simulink model "SistemaTotal"  (R2014b)
settings: Solver=FixedStepDiscrete  StartTime=0.0  StopTime=3000  RelTol=1e-3
undefined symbols (not defined in the file): M, T
settings Model: CovSFcnEnable=on  Creator=Afonso  LastModifiedBy=alunos
settings OptimizationCC: UseDivisionForNetSlopeComputation=off  SimCompilerOptimization=off
settings DebuggingCC: SolverPrmCheckMsg=none  FrameProcessingCompatibilityMsg=error
settings RTWCC: RTWCompilerOptimization=off

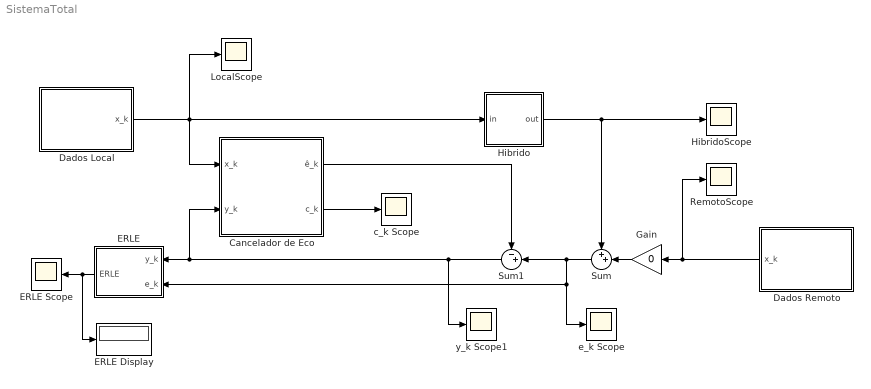
== system SistemaTotal ==
  Cancelador de Eco : Subsystem
  Dados Local : Subsystem
  Dados Remoto : Subsystem
  ERLE : Subsystem
  ERLE Display : Display
  ERLE Scope : Scope
      settings: TimeRange=1400  YMin=-1000  YMax=200  SaveName=ERLE
  Gain : Gain  Gain=0
  Hibrido : Subsystem
  HibridoScope : Scope
      settings: SaveName=Hibrido
  LocalScope : Scope
      settings: SaveName=Local
  RemotoScope : Scope
      settings: SaveName=Remoto
  Sum : Sum  Inputs=++|
  Sum1 : Sum  Inputs=-+|
  "c_k Scope " : Scope
      settings: SaveName=Coeficientes
  e_k Scope : Scope
      settings: SaveName=Eco
  y_k Scope1 : Scope
      settings: SaveName=Erro
  wires:
  Dados Local/1(x_k) -> LocalScope/1, Hibrido/1(in), Cancelador de Eco/1(x_k)
  Dados Remoto/1(x_k) -> RemotoScope/1, Gain/1
  Gain/1 -> Sum/2
  Hibrido/1(out) -> HibridoScope/1, Sum/1
  Cancelador de Eco/1(ê_k) -> Sum1/1
  ERLE/1(ERLE) -> ERLE Display/1, ERLE Scope/1
  Sum/1 -> e_k Scope/1, ERLE/2(e_k), Sum1/2
  Sum1/1 -> y_k Scope1/1, Cancelador de Eco/2(y_k), ERLE/1(y_k)
  Cancelador de Eco/2(c_k) -> "c_k Scope "/1

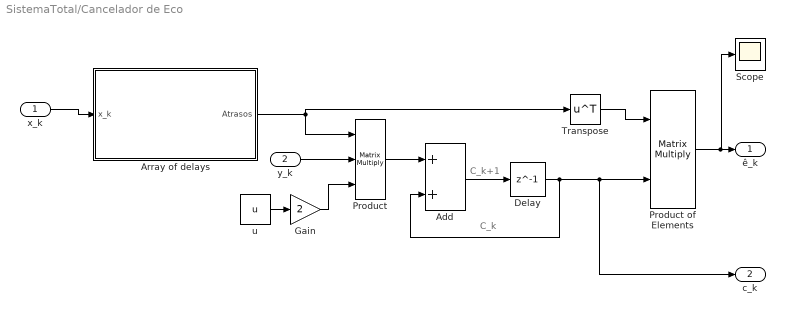
== system SistemaTotal/Cancelador de Eco ==
  note: C_k
  note: C_k+1
  x_k : Inport
  y_k : Inport  Port=2
  Add : Sum
  Array of delays : Subsystem
  Delay : Delay  DelayLength=1  SampleTime=T
  Gain : Gain  Gain=2
  Product : Product  Inputs=3  Multiplication=Matrix(*)
  Product of Elements : Product  Inputs=**  Multiplication=Matrix(*)
  Scope : Scope
  Transpose : Math  Operator=transpose  SaturateOnIntegerOverflow=on
  u : Constant  Value=u  SampleTime=T
  ê_k : Outport
  c_k : Outport  Port=2
  wires:
  y_k/1 -> Product/2
  u/1 -> Gain/1
  Gain/1 -> Product/3
  x_k/1 -> Array of delays/1(x_k)
  Product/1 -> Add/1
  Product of Elements/1 -> ê_k/1, Scope/1
  Add/1 -> Delay/1
  Delay/1 -> c_k/1, Product of Elements/2, Add/2
  Transpose/1 -> Product of Elements/1
  Array of delays/1(Atrasos) -> Product/1, Transpose/1

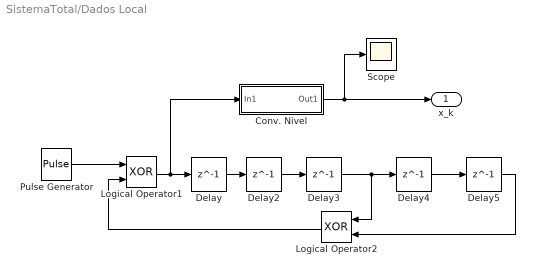
== system SistemaTotal/Dados Local ==
  Conv. Nivel : Subsystem
  Delay : Delay  DelayLength=1  SampleTime=T
  Delay{2..5} (4 alike) : Delay  DelayLength=1
  Logical Operator1 : Logic  Operator=XOR  AllPortsSameDT=off  OutDataTypeStr=boolean
  Logical Operator2 : Logic  Operator=XOR  AllPortsSameDT=off  OutDataTypeStr=boolean
  Pulse Generator : DiscretePulseGenerator  PulseType=Time based  Period=2*T  PulseWidth=50
  Scope : Scope
      settings: YMin=-1.5  YMax=1.5
  x_k : Outport
  wires:
  Delay2/1 -> Delay3/1
  Delay/1 -> Delay2/1
  Delay4/1 -> Delay5/1
  Delay3/1 -> Logical Operator2/1, Delay4/1
  Logical Operator2/1 -> Logical Operator1/2
  Delay5/1 -> Logical Operator2/2
  Logical Operator1/1 -> Conv. Nivel/1(In1), Delay/1
  Conv. Nivel/1(Out1) -> x_k/1, Scope/1
  Pulse Generator/1 -> Logical Operator1/1

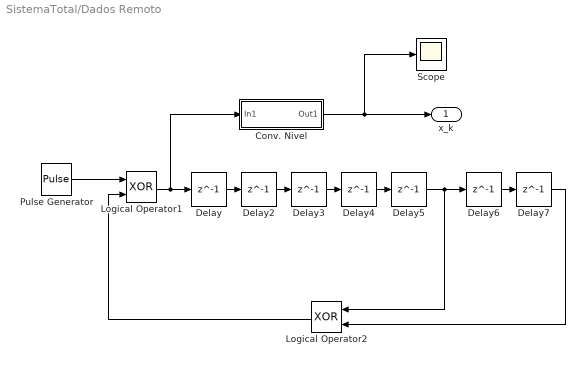
== system SistemaTotal/Dados Remoto ==
  Conv. Nivel : Subsystem
  Delay : Delay  DelayLength=1  SampleTime=T
  Delay{2..7} (6 alike) : Delay  DelayLength=1
  Logical Operator1 : Logic  Operator=XOR  AllPortsSameDT=off  OutDataTypeStr=boolean
  Logical Operator2 : Logic  Operator=XOR  AllPortsSameDT=off  OutDataTypeStr=boolean
  Pulse Generator : DiscretePulseGenerator  PulseType=Time based  Period=2*T  PulseWidth=50
  Scope : Scope
  x_k : Outport
  wires:
  Logical Operator1/1 -> Conv. Nivel/1(In1), Delay/1
  Delay4/1 -> Delay5/1
  Conv. Nivel/1(Out1) -> x_k/1, Scope/1
  Delay7/1 -> Logical Operator2/2
  Pulse Generator/1 -> Logical Operator1/1
  Logical Operator2/1 -> Logical Operator1/2
  Delay6/1 -> Delay7/1
  Delay5/1 -> Delay6/1, Logical Operator2/1
  Delay2/1 -> Delay3/1
  Delay/1 -> Delay2/1
  Delay3/1 -> Delay4/1

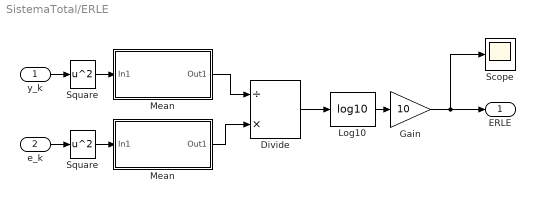
== system SistemaTotal/ERLE ==
  y_k : Inport
  e_k : Inport  Port=2
  Divide : Product  Inputs=/*
  Gain : Gain  Gain=10
  Log10 : Math  Operator=log10  SaturateOnIntegerOverflow=on
  Mean : Subsystem
  "Mean " : Subsystem
  Scope : Scope
  Square : Math  Operator=square  SaturateOnIntegerOverflow=on
  "Square " : Math  Operator=square  SaturateOnIntegerOverflow=on
  ERLE : Outport
  wires:
  e_k/1 -> "Square "/1
  y_k/1 -> Square/1
  "Square "/1 -> "Mean "/1(In1)
  "Mean "/1(Out1) -> Divide/2
  Log10/1 -> Gain/1
  Divide/1 -> Log10/1
  Gain/1 -> ERLE/1, Scope/1
  Mean/1(Out1) -> Divide/1
  Square/1 -> Mean/1(In1)

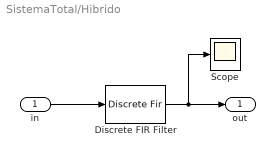
== system SistemaTotal/Hibrido ==
  in : Inport
  Discrete FIR Filter : DiscreteFir  Coefficients=[0 0.2 1 0.3 -0.4 -0.1 0.1 -0.05 -0.02 -0.01]  SampleTime=T
  Scope : Scope
  out : Outport
  wires:
  Discrete FIR Filter/1 -> out/1, Scope/1
  in/1 -> Discrete FIR Filter/1

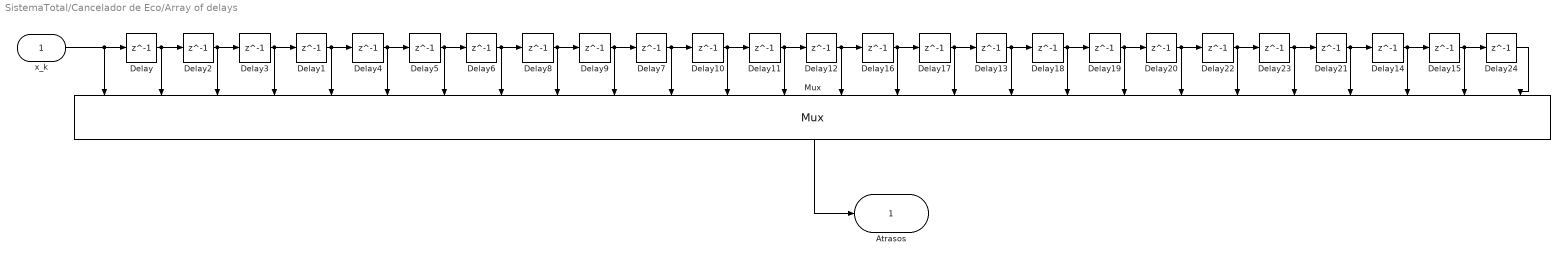
== system SistemaTotal/Cancelador de Eco/Array of delays ==
  x_k : Inport
  Delay : Delay  DelayLength=1  SampleTime=T
  Delay{1..24} (24 alike) : Delay  DelayLength=1
  Mux : Mux  Inputs=26
      settings: DisplayOption=signals
  Atrasos : Outport
  wires:
  Delay/1 -> Delay2/1, Mux/2
  Delay2/1 -> Mux/3, Delay3/1
  Delay11/1 -> Mux/13, Delay12/1
  Delay24/1 -> Mux/26
  Delay19/1 -> Delay20/1, Mux/19
  x_k/1 -> Delay/1, Mux/1
  Mux/1 -> Atrasos/1
  Delay15/1 -> Delay24/1, Mux/25
  Delay4/1 -> Mux/6, Delay5/1
  Delay1/1 -> Mux/5, Delay4/1
  Delay5/1 -> Mux/7, Delay6/1
  Delay12/1 -> Mux/14, Delay16/1
  Delay18/1 -> Mux/18, Delay19/1
  Delay16/1 -> Mux/15, Delay17/1
  Delay23/1 -> Delay21/1, Mux/22
  Delay17/1 -> Mux/16, Delay13/1
  Delay22/1 -> Delay23/1, Mux/21
  Delay14/1 -> Delay15/1, Mux/24
  Delay20/1 -> Delay22/1, Mux/20
  Delay13/1 -> Mux/17, Delay18/1
  Delay21/1 -> Delay14/1, Mux/23
  Delay8/1 -> Mux/9, Delay9/1
  Delay6/1 -> Mux/8, Delay8/1
  Delay10/1 -> Delay11/1, Mux/12
  Delay9/1 -> Delay7/1, Mux/10
  Delay7/1 -> Mux/11, Delay10/1
  Delay3/1 -> Mux/4, Delay1/1

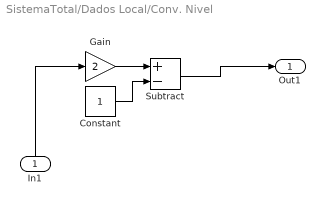
== system SistemaTotal/Dados Local/Conv. Nivel ==
  In1 : Inport
  Constant : Constant
  Gain : Gain  Gain=2
  Subtract : Sum  Inputs=+-
  Out1 : Outport
  wires:
  In1/1 -> Gain/1
  Constant/1 -> Subtract/2
  Gain/1 -> Subtract/1
  Subtract/1 -> Out1/1

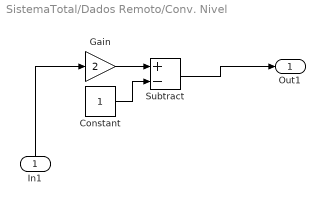
== system SistemaTotal/Dados Remoto/Conv. Nivel ==
  In1 : Inport
  Constant : Constant
  Gain : Gain  Gain=2
  Subtract : Sum  Inputs=+-
  Out1 : Outport
  wires:
  In1/1 -> Gain/1
  Constant/1 -> Subtract/2
  Gain/1 -> Subtract/1
  Subtract/1 -> Out1/1

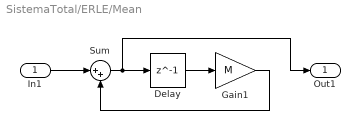
== system SistemaTotal/ERLE/Mean ==
  In1 : Inport
  Delay : Delay  DelayLength=1  SampleTime=T
  Gain1 : Gain  Gain=M
  Sum : Sum  Inputs=|++
  Out1 : Outport
  wires:
  Delay/1 -> Gain1/1
  Gain1/1 -> Sum/2
  In1/1 -> Sum/1
  Sum/1 -> Out1/1, Delay/1

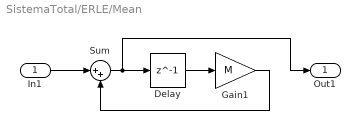
== system SistemaTotal/ERLE/Mean  ==
  In1 : Inport
  Delay : Delay  DelayLength=1  SampleTime=T
  Gain1 : Gain  Gain=M
  Sum : Sum  Inputs=|++
  Out1 : Outport
  wires:
  Delay/1 -> Gain1/1
  Gain1/1 -> Sum/2
  In1/1 -> Sum/1
  Sum/1 -> Out1/1, Delay/1
